simulink model "s6_template_2019a"  (R2019a)
settings: Solver=ode4  StartTime=0.0  StopTime=inf  FixedStep=P_sim_dt  RelTol=1e-3
InitFcn:
  | s6_data;
undefined symbols (not defined in the file or in its folder): CarInputsCmdForward, P_p_Bf, P_p_Br, P_p_Cf, P_p_Cr, P_p_Df, P_p_Dr, P_p_frontaxle_1, P_p_J, P_p_k, P_p_l, P_p_m, P_p_rearaxle_1, P_p_T, P_p_un_max, P_p_un_min, P_p_un_slow_max, P_p_un_slow_min, P_p_uTt, P_p_v_min
libraries: mad_lib_template x1
settings Model: EnablePacing=on  Creator=hmekiedj  LastModifiedBy=Daniel
settings DataIOCC: ReturnWorkspaceOutputs=off
settings DebuggingCC: ArithmeticOperatorsInVariantConditions=warning
settings SFSimCC: SimUseLocalCustomCode=off
settings RTWCC: RTWUseLocalCustomCode=off
settings CodeAppCC: StateflowObjectComments=on

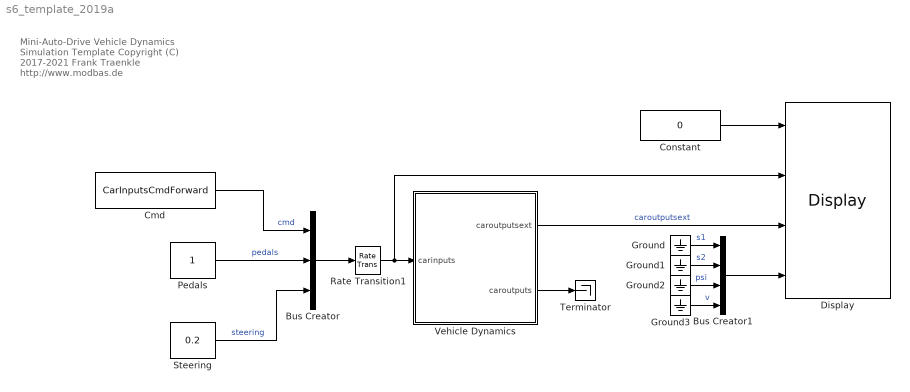
== system s6_template_2019a ==
  note: Mini-Auto-Drive
      | Vehicle Dynamics Simulation Template
      | Copyright (C) 2017-2021 Frank Traenkle
      | http://www.modbas.de
  Bus Creator : BusCreator  Inputs=3
  Bus Creator1 : BusCreator  Inputs=4
  Cmd : Constant  Value=CarInputsCmdForward  SampleTime=-1
  Constant : Constant  Value=0
  Display : mad_lib_template/Display  SystemSampleTime=-1  Latency=0  AutoFrameSizeCalculation=off
  Ground{,1..3} (4 alike) : Ground
  Pedals : Constant  SampleTime=-1
  Rate Transition1 : RateTransition
  Steering : Constant  Value=0.2  SampleTime=-1
  Terminator : Terminator
  Vehicle Dynamics : Subsystem
  wires:
  Bus Creator1/1 -> Display/4
  Ground/1 -> Bus Creator1/1  "s1"
  Ground1/1 -> Bus Creator1/2  "s2"
  Ground2/1 -> Bus Creator1/3  "psi"
  Ground3/1 -> Bus Creator1/4  "v"
  Vehicle Dynamics/1(caroutputsext) -> Display/3  "caroutputsext"
  Steering/1 -> Bus Creator/3  "steering"
  Rate Transition1/1 -> Display/2, Vehicle Dynamics/1(carinputs)
  Constant/1 -> Display/1
  Cmd/1 -> Bus Creator/1  "cmd"
  Vehicle Dynamics/2(caroutputs) -> Terminator/1
  Bus Creator/1 -> Rate Transition1/1
  Pedals/1 -> Bus Creator/2  "pedals"

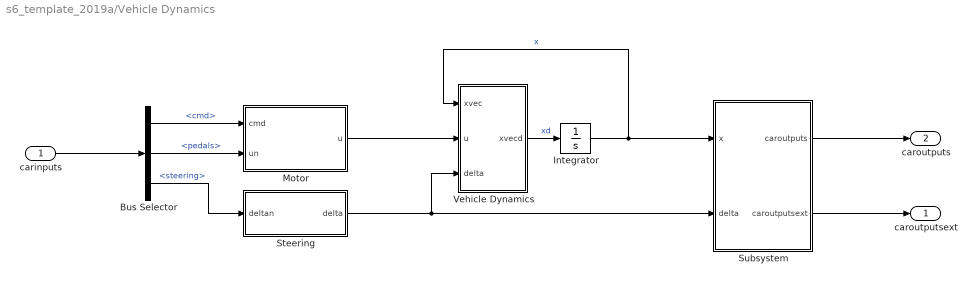
== system s6_template_2019a/Vehicle Dynamics ==
  carinputs : Inport
  Bus Selector : BusSelector  OutputSignals=cmd,pedals,steering
  Integrator : Integrator
  Motor : Subsystem
  Steering : Subsystem
  Subsystem : Subsystem
  Vehicle Dynamics : MATLAB Function  TreatAsAtomicUnit=on
  caroutputsext : Outport  VectorParamsAs1DForOutWhenUnconnected=off
  caroutputs : Outport  Port=2  VectorParamsAs1DForOutWhenUnconnected=off
  wires:
  carinputs/1 -> Bus Selector/1
  Bus Selector/2 -> Motor/2(un)  "<pedals>"
  Bus Selector/3 -> Steering/1(deltan)  "<steering>"
  Bus Selector/1 -> Motor/1(cmd)  "<cmd>"
  Steering/1(delta) -> Subsystem/2(delta), Vehicle Dynamics/3(delta)
  Integrator/1 -> Subsystem/1(x), Vehicle Dynamics/1(xvec)  "x"
  Subsystem/2(caroutputsext) -> caroutputsext/1
  Subsystem/1(caroutputs) -> caroutputs/1
  Motor/1(u) -> Vehicle Dynamics/2(u)
  Vehicle Dynamics/1(xvecd) -> Integrator/1  "xd"

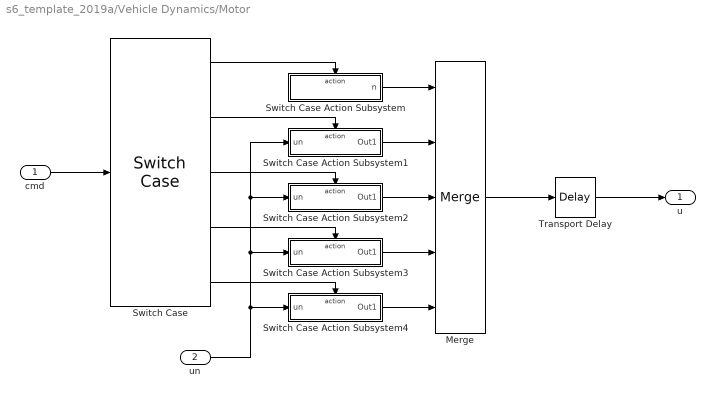
== system s6_template_2019a/Vehicle Dynamics/Motor ==
  cmd : Inport
  un : Inport  Port=2
  Merge : Merge  Inputs=5
  Switch Case : SwitchCase  CaseConditions={0,1,2,3}
  Switch Case Action Subsystem : Subsystem  TreatAsAtomicUnit=on
  Switch Case Action Subsystem1 : Subsystem  TreatAsAtomicUnit=on
  Switch Case Action Subsystem2 : Subsystem  TreatAsAtomicUnit=on
  Switch Case Action Subsystem3 : Subsystem  TreatAsAtomicUnit=on
  Switch Case Action Subsystem4 : Subsystem  TreatAsAtomicUnit=on
  Transport Delay : TransportDelay  DelayTime=P_p_uTt
  u : Outport
  wires:
  cmd/1 -> Switch Case/1
  un/1 -> Switch Case Action Subsystem1/1(un), Switch Case Action Subsystem2/1(un), Switch Case Action Subsystem3/1(un), Switch Case Action Subsystem4/1(un)
  Switch Case Action Subsystem/1(n) -> Merge/1
  Switch Case Action Subsystem1/1(Out1) -> Merge/2
  Switch Case Action Subsystem2/1(Out1) -> Merge/3
  Switch Case Action Subsystem3/1(Out1) -> Merge/4
  Switch Case Action Subsystem4/1(Out1) -> Merge/5
  Merge/1 -> Transport Delay/1
  Transport Delay/1 -> u/1
  Switch Case/1 -> Switch Case Action Subsystem/Action
  Switch Case/2 -> Switch Case Action Subsystem1/Action
  Switch Case/3 -> Switch Case Action Subsystem2/Action
  Switch Case/4 -> Switch Case Action Subsystem3/Action
  Switch Case/5 -> Switch Case Action Subsystem4/Action

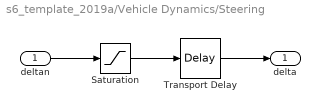
== system s6_template_2019a/Vehicle Dynamics/Steering ==
  deltan : Inport
  Saturation : Saturate  UpperLimit=P_p_un_max  LowerLimit=P_p_un_min  LinearizeAsGain=off
  Transport Delay : TransportDelay  DelayTime=P_p_uTt
  delta : Outport
  wires:
  deltan/1 -> Saturation/1
  Saturation/1 -> Transport Delay/1
  Transport Delay/1 -> delta/1

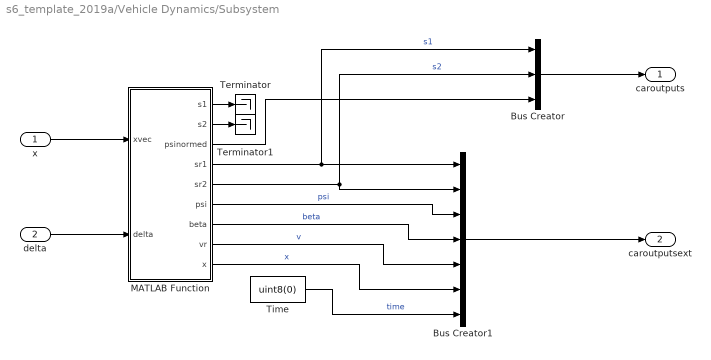
== system s6_template_2019a/Vehicle Dynamics/Subsystem ==
  x : Inport
  delta : Inport  Port=2
  Bus Creator : BusCreator  Inputs=3
  Bus Creator1 : BusCreator  Inputs=7  OutDataTypeStr=Bus: CAROUTPUTSEXT  NonVirtualBus=on
  MATLAB Function : MATLAB Function  TreatAsAtomicUnit=on
  Terminator : Terminator
  Terminator1 : Terminator
  Time : Constant  Value=uint8(0)
  caroutputs : Outport
  caroutputsext : Outport  Port=2
  wires:
  MATLAB Function/8(vr) -> Bus Creator1/5  "v"
  MATLAB Function/6(psi) -> Bus Creator1/3  "psi"
  MATLAB Function/5(sr2) -> Bus Creator/2, Bus Creator1/2  "s2"
  MATLAB Function/7(beta) -> Bus Creator1/4  "beta"
  MATLAB Function/9(x) -> Bus Creator1/6  "x"
  Time/1 -> Bus Creator1/7  "time"
  MATLAB Function/4(sr1) -> Bus Creator/1, Bus Creator1/1  "s1"
  Bus Creator1/1 -> caroutputsext/1
  x/1 -> MATLAB Function/1(xvec)
  delta/1 -> MATLAB Function/2(delta)
  Bus Creator/1 -> caroutputs/1
  MATLAB Function/3(psinormed) -> Bus Creator/3
  MATLAB Function/1(s1) -> Terminator/1
  MATLAB Function/2(s2) -> Terminator1/1

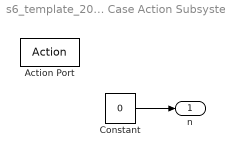
== system s6_template_2019a/Vehicle Dynamics/Motor/Switch Case Action Subsystem ==
  Action Port : ActionPort
  Constant : Constant  Value=0
  n : Outport
  wires:
  Constant/1 -> n/1

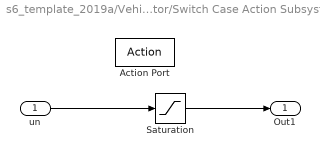
== system s6_template_2019a/Vehicle Dynamics/Motor/Switch Case Action Subsystem1 ==
  un : Inport
  Action Port : ActionPort
  Saturation : Saturate  UpperLimit=P_p_un_max  LowerLimit=0
  Out1 : Outport
  wires:
  un/1 -> Saturation/1
  Saturation/1 -> Out1/1

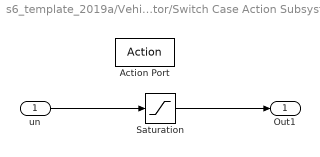
== system s6_template_2019a/Vehicle Dynamics/Motor/Switch Case Action Subsystem2 ==
  un : Inport
  Action Port : ActionPort
  Saturation : Saturate  UpperLimit=0  LowerLimit=P_p_un_min
  Out1 : Outport
  wires:
  un/1 -> Saturation/1
  Saturation/1 -> Out1/1

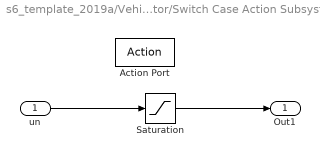
== system s6_template_2019a/Vehicle Dynamics/Motor/Switch Case Action Subsystem3 ==
  un : Inport
  Action Port : ActionPort
  Saturation : Saturate  UpperLimit=P_p_un_slow_max  LowerLimit=P_p_un_slow_min
  Out1 : Outport
  wires:
  un/1 -> Saturation/1
  Saturation/1 -> Out1/1

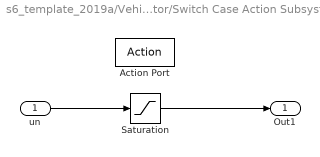
== system s6_template_2019a/Vehicle Dynamics/Motor/Switch Case Action Subsystem4 ==
  un : Inport
  Action Port : ActionPort
  Saturation : Saturate  UpperLimit=P_p_un_max  LowerLimit=P_p_un_min
  Out1 : Outport
  wires:
  un/1 -> Saturation/1
  Saturation/1 -> Out1/1

== matlab function s6_template_2019a/Vehicle Dynamics/Subsystem/MATLAB Function ==
  data: s1 output; s2 output; xvec input; delta input; psinormed output; sr1 output; sr2 output; psi output; beta output; vr output; x output; P_p_rearaxle_1 parameter; P_p_v_min parameter; P_p_l parameter
function [s1, s2, psinormed, sr1, sr2, psi, beta, vr, x] = outputs(xvec, delta, P_p_rearaxle_1, P_p_v_min, P_p_l)

temp2 = zeros(4,1);
temp2 = xvec;

vc1 = temp2(1);
s1 = temp2(2);
s2 = temp2(3);
psi = temp2(4);
x = temp2(7);

psinormed = mod(psi, 2*pi);
if psinormed > pi
    psinormed = psinormed - 2*pi;
end
beta = 0;
sr1 = s1 - P_p_rearaxle_1 * cos(psi);
sr2 = s2 - P_p_rearaxle_1 * sin(psi);
vr = vc1;
end

== matlab function s6_template_2019a/Vehicle Dynamics/Vehicle Dynamics ==
  data: xvec input; u input; delta input; xvecd output; P_p_Br parameter; P_p_Bf parameter; P_p_Cr parameter; P_p_Cf parameter; P_p_Dr parameter; P_p_Df parameter; P_p_rearaxle_1 parameter; P_p_frontaxle_1 parameter; P_p_m parameter; P_p_J parameter; P_p_k parameter; P_p_T parameter; P_p_v_min parameter; P_p_l parameter
function xvecd = dynamics(xvec, u, delta, P_p_Br, P_p_Bf, P_p_Cr, P_p_Cf, P_p_Dr, P_p_Df, ...
    P_p_rearaxle_1, P_p_frontaxle_1, P_p_m, P_p_J, P_p_k, P_p_T, P_p_v_min, P_p_l)

temp = zeros(7,1);
temp = xvec;

vc1 = temp(1);
psi = temp(4);
psid = temp(5);
vc2 = temp(6);

if abs(vc1) > P_p_v_min % avoid model singularity at zero speed
    %% bicycle model with Magic Tire
    spsi = sin(psi);
    cpsi = cos(psi);
    sdelta = sin(delta);
    cdelta = cos(delta);
    
    % wheel slip angles
    alphaf = -atan2(vc2 + P_p_frontaxle_1 * psid, vc1) + delta;
    alphar = -atan2(vc2 - P_p_rearaxle_1 * psid, vc1);
    % wheel forces
    Ff = P_p_Df * sin(P_p_Cf * atan(P_p_Bf * alphaf));
    Fr = P_p_Dr * sin(P_p_Cr * atan(P_p_Br * alphar));    
    % logitudinal dynamics (momentum balance)
    vc1d = (-Ff * sdelta + P_p_m * vc2 * psid) / P_p_m ...
            - vc1/P_p_T + P_p_k/P_p_T * u;
    % kinematics
    s1d = vc1 * cpsi - vc2 * spsi;
    s2d = vc1 * spsi + vc2 * cpsi;
    % rotational dynamics (moment of momentum balance)
    psidd = (Ff * P_p_frontaxle_1 * cdelta - Fr * P_p_rearaxle_1) / P_p_J;
    % lateral dynamics (momentum balance)
    vc2d = (Ff * cdelta + Fr - P_p_m * vc1 * psid)/P_p_m;
    % driven arc length of rear axle center
    xd = vc1;
else % near zero speed
    %% longitudinal dynamics of rear axle
    a = P_p_rearaxle_1;
    l = P_p_l;
    spsi = sin(psi);
    cpsi = cos(psi);
    tdelta = tan(delta);
    vc2 = a/l * vc1 * tdelta;
    vc1d = (-vc1 + P_p_k * u) / P_p_T; % -(a^2+P_p_J/P_p-m)/l^2*vc1*tdelta*deltad
    s1d = vc1 * cpsi - vc2 * spsi;
    s2d = vc1 * spsi + vc2 * cpsi;
    psid = vc1 / l * tdelta;
    psidd = 0; % vc1d / l * tdelta + vc1/l * deltad * (1 + tdelta*delta)
    vc2d = 0 ; % a * psidd;
    xd = vc1;
end
    
xvecd = [ vc1d; s1d; s2d; psid; psidd; vc2d; xd ];
end
